simulink model "estimator_noise"  (R2015b)
settings: Solver=ode45  StartTime=0.0  StopTime=10.0  RelTol=1e-3
values from neighbouring files (symbols this model uses):
  A = -1    [estimator.m]    (also in main_quad.m = jacobian(1:12,1:12); two_tanks_tracking_controller.m = [-0.0891 0.0891)
  B = 1    [estimator.m]    (also in main_quad.m = jacobian(1:12,13:16); two_tanks_tracking_controller.m = [14.0845 0)
  C = 1    [estimator.m]    (also in main_quad.m = [eye(3) zeros(3,9); two_tanks_tracking_controller.m = [1 0)
  L1 = acker(A',C',-10)'    [estimator.m]
  L2 = acker(A',C',-2)'    [estimator.m]
  x0 = 1    [estimator.m]
  xest = 0    [estimator.m]
settings Model: Creator=Mauricio  LastModifiedBy=Mauricio
settings DataIOCC: SaveFormat=Array  SignalLoggingSaveFormat=ModelDataLogs
settings OptimizationCC: ExpressionDepthLimit=2147483647
settings DebuggingCC: UnderspecifiedInitializationDetection=Classic  MergeDetectMultiDrivingBlocksExec=none  SolverPrmCheckMsg=warning  FcnCallInpInsideContextMsg=UseLocalSettings  StateNameClashWarn=warning
settings HardwareCC: ProdBitPerPointer=32  ProdLargestAtomicFloat=None  ProdIntDivRoundTo=Undefined  ProdEndianess=Unspecified  ProdWordSize=32  ProdHWDeviceType=32-bit Generic
settings GRTTargetCC: CombineOutputUpdateFcns=off  GRTInterface=on
settings ConfigComp: CovModelRefEnable=Off

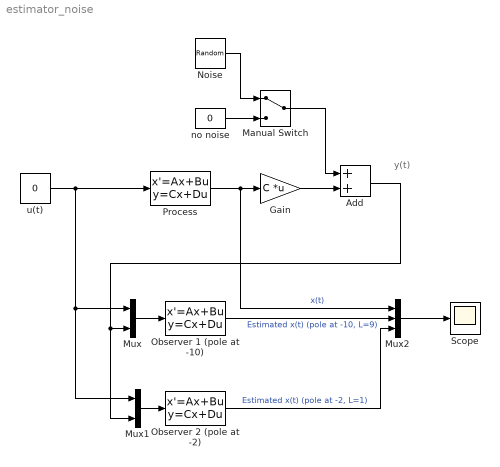
== system estimator_noise ==
  note: y(t)
  Add : Sum
  Gain : Gain  Gain=C  Multiplication=Matrix(K*u)
  Manual Switch : ManualSwitch
  Mux : Mux  Inputs=2
  Mux1 : Mux  Inputs=2
  Mux2 : Mux  Inputs=3
  Noise : RandomNumber  Variance=0.01  SampleTime=0.1
  Observer 1 (pole at -10) : StateSpace  A=A-L1*C  B=[B L1]  D=[0 0]  X0=xest
  Observer 2 (pole at -2) : StateSpace  A=A-L2*C  B=[B L2]  D=[0 0]  X0=xest
  Process : StateSpace  A=A  B=B  D=0  X0=x0
  Scope : Scope
  no noise : Constant  Value=0
  u(t) : Constant  Value=0
  wires:
  u(t)/1 -> Process/1, Mux/1, Mux1/1
  Process/1 -> Gain/1, Mux2/1  "x(t)"
  Gain/1 -> Add/2
  Add/1 -> Mux/2, Mux1/2
  Manual Switch/1 -> Add/1
  no noise/1 -> Manual Switch/2
  Noise/1 -> Manual Switch/1
  Mux/1 -> Observer 1 (pole at -10)/1
  Mux1/1 -> Observer 2 (pole at -2)/1
  Observer 1 (pole at -10)/1 -> Mux2/2  "Estimated x(t) (pole at -10, L=9)"
  Observer 2 (pole at -2)/1 -> Mux2/3  "Estimated x(t) (pole at -2, L=1)"
  Mux2/1 -> Scope/1
